simulink model "Fahrzeugbeschleunigung"  (Simulink 7.1)
settings: Solver=ode45  StartTime=0.0  StopTime=10.0  RelTol=1e-3
settings Model: Creator=Meisel  LastModifiedBy=Meisel

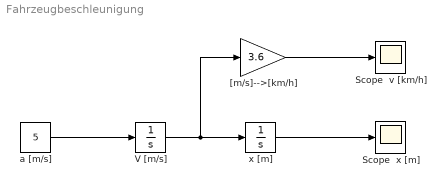
== system Fahrzeugbeschleunigung ==
  Scope  v [km/h] : Scope
  Scope  x [m] : Scope
  V [m/s] : Integrator  InitialCondition=50/3.6
  "[m/s]-->[km/h]" : Gain  Gain=3.6  ParameterDataType=sfix(16)  ParameterScaling=2^0  OutDataType=sfix(16)  OutScaling=2^0
  a [m/s] : Constant  Value=5  OutDataType=sfix(16)  OutScaling=2^0
  x [m] : Integrator
  wires:
  a [m/s]/1 -> V [m/s]/1
  V [m/s]/1 -> x [m]/1, "[m/s]-->[km/h]"/1
  x [m]/1 -> Scope  x [m]/1
  "[m/s]-->[km/h]"/1 -> Scope  v [km/h]/1
